simulink model "UtoH"  (R2020b)
settings: Solver=VariableStepAuto  StartTime=0.0  StopTime=300  RelTol=1e-3
undefined symbols (not defined in the file): National_Instruments, PCIe
libraries: sldrtlib x2, dspstat3 x1
settings Model: Creator=EAL  LastModifiedBy=EAL

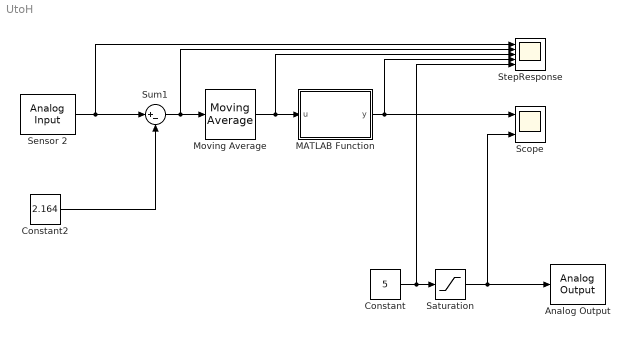
== system UtoH ==
  Analog Output : sldrtlib/Analog Output  SampleTime=0.1  MaxMissedTicks=10  ShowMissedTicks=off  YieldWhenWaiting=off  DrvName=National_Instruments/PCIe-6321  DrvAddress=4294967295  DrvOptions=[0 0 0 0 0 0 0]  Channels=1  RangeMode=1  VoltRange=1  InitialValue=[]  FinalValue=[]
      settings: AttributesFormatString=National Instruments\nPCIe-6321 [auto]
  Constant : Constant  Value=5
  Constant2 : Constant  Value=2.164
  MATLAB Function : MATLAB Function  TreatAsAtomicUnit=on
  Moving Average : dspstat3/Moving Average  Method=Sliding window  ForgettingFactorPort=off  SpecifyWindowLength=on  WindowLength=6  ForgettingFactor=0.9  SimulateUsing=Code generation
  Saturation : Saturate  UpperLimit=5  LowerLimit=0
  Scope : Scope  NumInputPorts=2
  Sensor 2 : sldrtlib/Analog Input  SampleTime=0.1  MaxMissedTicks=10  ShowMissedTicks=off  YieldWhenWaiting=off  DrvName=National_Instruments/PCIe-6321  DrvAddress=4294967295  DrvOptions=[0 0 0 0 0 0 0]  Channels=3  RangeMode=1  VoltRange=1  DataType=1
      settings: AttributesFormatString=National Instruments\nPCIe-6321 [auto]
  StepResponse : Scope  NumInputPorts=5
  Sum1 : Sum  Inputs=|+-
  wires:
  Constant2/1 -> Sum1/2
  Saturation/1 -> Scope/2, Analog Output/1
  Sensor 2/1 -> StepResponse/1, Sum1/1
  MATLAB Function/1(y) -> StepResponse/4, Scope/1
  Sum1/1 -> StepResponse/2, Moving Average/1
  Moving Average/1 -> StepResponse/3, MATLAB Function/1(u)
  Constant/1 -> StepResponse/5, Saturation/1

== matlab function UtoH/MATLAB Function ==
  data: u input; y output
function y = fcn(u)

y = 1.192708333333333e+02 * u + 3.744791666666675;
